simulink model "TST_DuringActionTest"  (Simulink 10.0)
settings: Solver=FixedStepDiscrete  StartTime=0.0  StopTime=10.0  FixedStep=0.02  RelTol=1e-3  EnableMultiTasking=on
settings Model: Creator=kharthforeign  LastModifiedBy=unknown
settings DataIOCC: LimitDataPoints=on  SignalLoggingSaveFormat=ModelDataLogs  SaveOutput=off  SignalLogging=off  SaveTime=off
settings OptimizationCC: BlockReduction=off  ConditionallyExecuteInputs=off  OptimizeBlockIOStorage=off  BufferReuse=off  GlobalBufferReuse=off  ExpressionFolding=off  ExpressionDepthLimit=2147483647  LocalBlockOutputs=off  InitFltsAndDblsToZero=on  OptimizeDataStoreBuffers=off  BusAssignmentInplaceUpdate=off
settings DebuggingCC: SolverPrmCheckMsg=warning  FcnCallInpInsideContextMsg=warning  StateNameClashWarn=warning
settings SFSimCC: SimParseCustomCode=off
settings RTWCC: GenCodeOnly=on
settings GRTTargetCC: GeneratePreprocessorConditionals=Disable all
settings ConfigComp: CovExternalEMLEnable=off

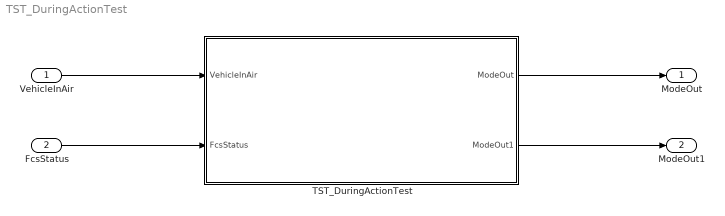
== system TST_DuringActionTest ==
  VehicleInAir : Inport  OutDataTypeStr=boolean  PortDimensions=1
  FcsStatus : Inport  Port=2  OutDataTypeStr=Bus: FCS_FlightControlSystem_Status
  TST_DuringActionTest : Subsystem  TreatAsAtomicUnit=on
  ModeOut : Outport  OutDataTypeStr=int32  PortDimensions=1
  ModeOut1 : Outport  Port=2  OutDataTypeStr=int32  PortDimensions=1
  wires:
  VehicleInAir/1 -> TST_DuringActionTest/1(VehicleInAir)
  FcsStatus/1 -> TST_DuringActionTest/2(FcsStatus)
  TST_DuringActionTest/1(ModeOut) -> ModeOut/1
  TST_DuringActionTest/2(ModeOut1) -> ModeOut1/1

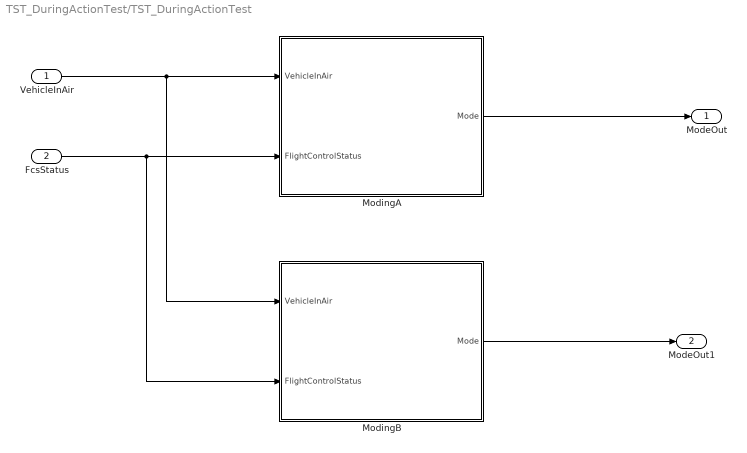
== system TST_DuringActionTest/TST_DuringActionTest ==
  VehicleInAir : Inport  OutDataTypeStr=boolean  PortDimensions=1
  FcsStatus : Inport  Port=2  OutDataTypeStr=Bus: FCS_FlightControlSystem_Status
  ModingA : Stateflow chart  TreatAsAtomicUnit=on
  ModingB : Stateflow chart  TreatAsAtomicUnit=on
  ModeOut : Outport  OutDataTypeStr=int32  PortDimensions=1
  ModeOut1 : Outport  Port=2  OutDataTypeStr=int32  PortDimensions=1
  wires:
  FcsStatus/1 -> ModingA/2(FlightControlStatus), ModingB/2(FlightControlStatus)
  VehicleInAir/1 -> ModingA/1(VehicleInAir), ModingB/1(VehicleInAir)
  ModingA/1(Mode) -> ModeOut/1
  ModingB/1(Mode) -> ModeOut1/1

== stateflow chart TST_DuringActionTest/ModingA ==
  state TopStateA
    during:
    Mode = int32(111);
    state Autoland
      entry:
      Mode = int32(3);
      during:
      Mode = int32(-3);
    state Off
      entry:
      Mode = int32(1);
    state Launch
      entry:
      Mode = int32(2);
    (default) -> Off
    Off -> Launch : [(FlightControlStatus.PressureAltitude_Ft < 500.0) && (~VehicleInAir)]
    Launch -> Autoland : [(FlightControlStatus.PressureAltitude_Ft > 1500.0) || VehicleInAir]
  state TopStateB
    during:
    Mode = int32(222);
  (default) -> TopStateA
  TopStateA -> TopStateB : [Mode >= int32(123)]
  data: VehicleInAir input boolean; Mode output int32; FlightControlStatus input FCS_FlightControlSystem_Status

== stateflow chart TST_DuringActionTest/ModingB ==
  state TopStateA
    during:
    Mode = int32(111);
    state Autoland
      entry:
      Mode = int32(3);
      during:
      Mode = int32(-3);
    state Off
      entry:
      Mode = int32(1);
    state Launch
      entry:
      Mode = int32(2);
      during:
      Mode = int32(-2);
    (default) -> Off
    Off -> Launch : [(FlightControlStatus.PressureAltitude_Ft < 500.0) && (~VehicleInAir)]
    Launch -> Autoland [order 1] : [FlightControlStatus.PressureAltitude_Ft > 1500.0]
  state TopStateB
    during:
    Mode = int32(222);
  (default) -> TopStateA
  TopStateA -> TopStateB : [Mode >= int32(123)]
  Launch -> TopStateB [order 2] : [VehicleInAir]
  TopStateB -> TopStateA
  data: VehicleInAir input boolean; Mode output int32; FlightControlStatus input FCS_FlightControlSystem_Status
